simulink model "Line Following"  (R2023a)
settings: Solver=FixedStepDiscrete  StartTime=0.0  StopTime=30  FixedStep=0.01  RelTol=1e-3
values from neighbouring files (symbols this model uses):
  InputPWM = [-127 -126 -125 -124 -123 -122 -121 -120 -119 -118 -117 -116 ... (173 elements, 1x173)]    [ROBOT_WORKSPACE.mat]
  WheelSpeed = [-12.5105278523 -12.3751973908 -12.2398669292 -12.1045364677 -11.9692060062 -11.8338755446 -11.6985450831 -11.5632146215 -11.42788416 -11.2925536985 -11.1572232369 -11.0218927754 ... (173 elements, 1x173)]    [ROBOT_WORKSPACE.mat]
libraries: mobileRoboticsTrainingLib x5
settings Model: Creator=nuvitdemirtas  LastModifiedBy=nuvitdemirtas

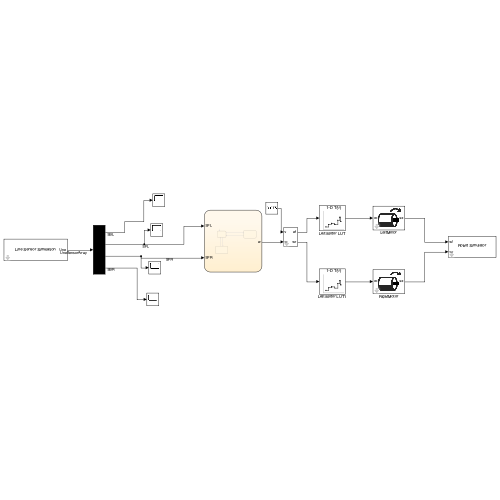
[thumbnail: Simulink's stored preview of the top-level diagram]
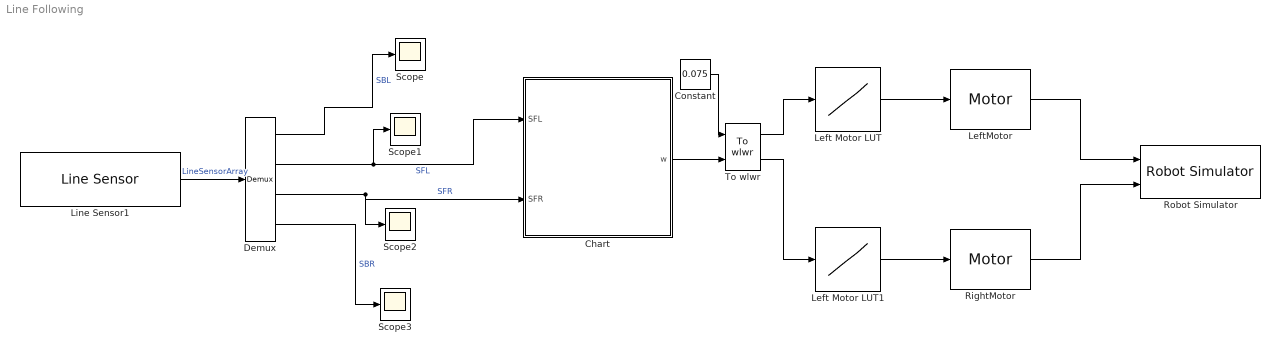
== system Line Following ==
  Chart : Stateflow chart  TreatAsAtomicUnit=on
      settings: PortSchema="{\"entries\":[{\"content\":{\"sides\":[{\"content\":{\"connectorIds\":[\"In2\",\"In1\"]},\"type\":\"ConnectorPlacement.EquallySpacedRectSide\",\"uuid\":\"3b08c9f5-f3e7-4190-8c9e-e5c4b273b76c\"},{\"content\":{\"connectorIds\":[\"Out1\"],\"side\":\"RIGHT\"},\"type\":\"ConnectorPlacement.EquallySpacedRectSide\",\"uuid\":\"91158a50-9984-4409-9676-111dc7610217\"},{\"content\":{\"side\":\"TOP\"},\"type\":\"ConnectorPlacement.EquallySpacedRectSide\",\"uuid\":\"e43f7616-6a00-4e82-aaba-e999a0c0a235\"}]},\"type\":\"ConnectorPlacement.EquallySpacedConnector\",\"uuid\":\"4b7d5f21-cf1e-4123-a6bd-16491044a199\"}],\"packageUris\":[\"http://schema.mathworks.com/mf0/Connector/R2020b\"],\"version\":\"1.0\"}"
  Constant : Constant  Value=0.075
  Demux : Demux
  Left Motor LUT : Lookup_n-D  NumberOfTableDimensions=1  BreakpointsForDimension1=WheelSpeed  Table=InputPWM  InterpMethod=Nearest  ExtrapMethod=Clip  InternalRulePriority=Speed  RndMeth=Simplest
  Left Motor LUT1 : Lookup_n-D  NumberOfTableDimensions=1  BreakpointsForDimension1=WheelSpeed  Table=InputPWM  InterpMethod=Nearest  ExtrapMethod=Clip  InternalRulePriority=Speed  RndMeth=Simplest
  LeftMotor : mobileRoboticsTrainingLib/Motor  motorPlant=wheelMotorModel  sensorType=Speed
      settings: SourceProductName=Mobile Robotics Training Library
  Line Sensor1 : mobileRoboticsTrainingLib/Line Sensor  mapVariable=mapForSim  envVal=1  lineVal=0  sensOff=[0.0643 0.0354; 0.0675 0.005; 0.0675 -0.005; 0.0643 -0.0354]
      link override Switch: Threshold=0
      settings: SourceProductName=Mobile Robotics Training Library
  RightMotor : mobileRoboticsTrainingLib/Motor  motorPlant=wheelMotorModel  sensorType=Speed
      settings: SourceProductName=Mobile Robotics Training Library
  Robot Simulator : mobileRoboticsTrainingLib/Robot Simulator  Priority=99  mapVar=mapForSim  startX=0.5862  startY=0.089122  startTheta=90  axleLength=axleLength  wheelR=wheelR
  Scope{,1..3} (4 alike) : Scope
  To wlwr : mobileRoboticsTrainingLib/To wlwr  axleLength=0.1  wheelR=0.05
  wires:
  To wlwr/2 -> Left Motor LUT1/1
  To wlwr/1 -> Left Motor LUT/1
  Left Motor LUT/1 -> LeftMotor/1
  RightMotor/1 -> Robot Simulator/2
  Left Motor LUT1/1 -> RightMotor/1
  LeftMotor/1 -> Robot Simulator/1
  Line Sensor1/1 -> Demux/1  "LineSensorArray"
  Demux/1 -> Scope/1  "SBL"
  Demux/3 -> Chart/1(SFR), Scope2/1  "SFR"
  Demux/4 -> Scope3/1  "SBR"
  Demux/2 -> Chart/2(SFL), Scope1/1  "SFL"
  Chart/1(w) -> To wlwr/2
  Constant/1 -> To wlwr/1

== stateflow chart Line Following/Chart ==
  state CORRECT_right
    entry:
    w = -1;
  state perfect
    entry:
    w = 0;
  state CORRECT_left
    entry:
    w = 1;
  (default) -> perfect
  perfect -> CORRECT_right [order 1] : [SFR == 0 && SFL ==1]
  CORRECT_right -> perfect : [SFR == 0 && SFL ==0]
  CORRECT_left -> perfect : [SFR == 0 && SFL ==0]
  perfect -> CORRECT_left [order 2] : [SFR == 1 && SFL ==0]
  data: w output; SFR input; SFL input
